simulink model "qpBoxFcnSim_14b"  (R2014b)
settings: Solver=FixedStepDiscrete  SolverMode=SingleTasking  StartTime=0.0  StopTime=10.0  FixedStep=0.1  RelTol=1e-3
settings Model: CovMetricSettings=dwe  CovHtmlReporting=off  covSaveCumulativeToWorkspaceVar=off  CovSaveSingleToWorkspaceVar=off  CovExternalEMLEnable=on  CovSFcnEnable=on  Creator=thomasbruen  LastModifiedBy=BRUEN_T
settings DataIOCC: LimitDataPoints=off  SaveFormat=StructureWithTime
settings DebuggingCC: SolverPrmCheckMsg=none  FrameProcessingCompatibilityMsg=error  SFUnexpectedBacktrackingDiag=error  SFNoUnconditionalDefaultTransitionDiag=error
settings HardwareCC: ProdBitPerPointer=64  ProdLargestAtomicFloat=Float  ProdIntDivRoundTo=Zero  ProdEndianess=LittleEndian  ProdHWDeviceType=Specified
settings ModelReferenceCC: PropagateSignalLabelsOutOfModel=on
settings GRTTargetCC: TargetLangStandard=C99 (ISO)  GeneratePreprocessorConditionals=Use local settings

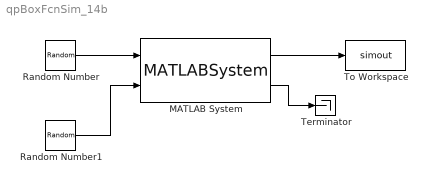
== system qpBoxFcnSim_14b ==
  MATLAB System : MATLABSystem  System=qpBoxFcnTest  N=10  tolFun=1e-8  gamma=0.8  maxIter=25  lb=lb  ub=ub  SimulateUsing=Interpreted execution
      mask Type: qpBoxFcnTest
      mask Display:
      | disp('qpBoxFcnTest');
      | port_label('output',1,'u');
      | port_label('output',2,'statusFlag');
  Random Number : RandomNumber  Mean=5  SampleTime=0.1
  Random Number1 : RandomNumber  Variance=2  SampleTime=0.1
  Terminator : Terminator
  To Workspace : ToWorkspace  VariableName=simout  SampleTime=-1
  wires:
  MATLAB System/2 -> Terminator/1
  MATLAB System/1 -> To Workspace/1
  Random Number/1 -> MATLAB System/1
  Random Number1/1 -> MATLAB System/2
